simulink model "attack_decay_filter_optimized"  (R2020b)
settings: Solver=FixedStepAuto  StartTime=0.0  StopTime=stopTime  RelTol=1e-3
values from neighbouring files (symbols this model uses):
  buf_a = 65 .* ones(num_bands,1)    [modelparameters.m]
  buf_d = 65 .* ones(num_bands,1)    [modelparameters.m]
  num_bands = 8    [modelparameters.m]
libraries: simulink x1
settings Model: Creator=conno  LastModifiedBy=conno
settings DataIOCC: ReturnWorkspaceOutputs=off
settings ModelReferenceCC: ModelReferenceNumInstancesAllowed=Single

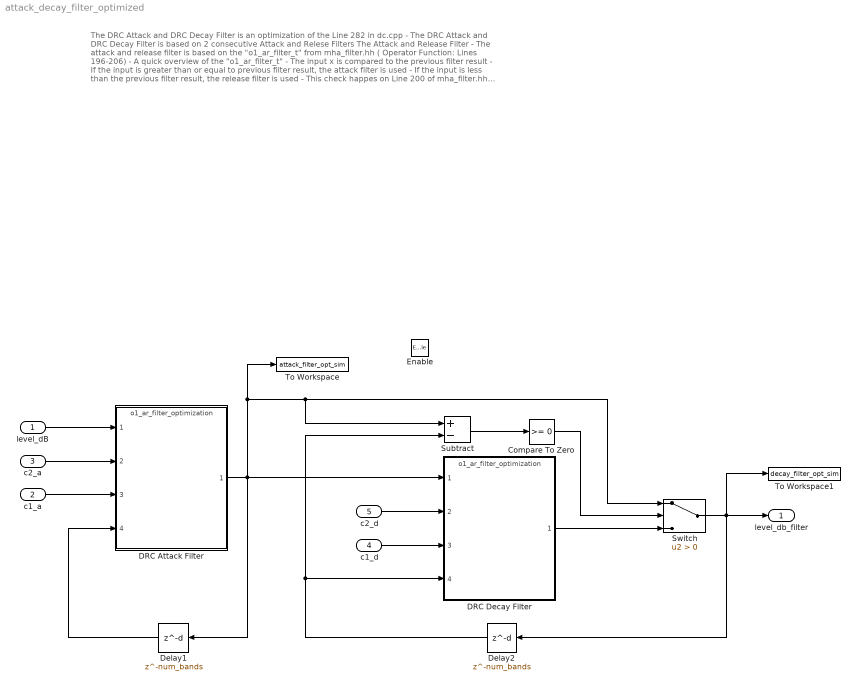
== system attack_decay_filter_optimized ==
  note: The DRC Attack and DRC Decay Filter is an optimization of the Line 282 in dc.cpp
      | - The DRC Attack and DRC Decay Filter is based on 2 consecutive Attack and Relese Filters
      | The Attack and Release Filter
      | - The attack and release filter is based on the "o1_ar_filter_t" from mha_filter.hh ( Operator Function: Lines 196-206)
      | - A quick overview of the "o1_ar_filter_t"
      | - The input x is compared to the previous filter result
      | - If the input is greater than or equal to previous filter result, the attack filter is used
      | - If the input is less than the previous filter result, the release filter is used
      | - This check happes on Line 200 of mha_filter.hh
      | Attack and Decay Filter Implementation in dc.cpp
      | - The DRC Attack Filter is a simplification of the "o1_ar_filter_t"
      | - The attack and release coefficients are the same - Lines 448-452 of mha_filter.cpp
      | - This mitigates the if statement (Line 200) of the "o1_ar_filter_t"
      | - The DRC Decay Filter is a simplifcation of the "o1_ar_filter_t" - Lines 505-509 of mha_filter.cpp
      | - The attack time constant is equal to 0
      | - c1 = 0
      | - c2 = 1
      | - The release coefficients are computed using the decay time constant
      | Simulink Optimization
      | - The DRC Attack Filter is simplified by using a single set of coefficients
      | - The result of the DRC Attack Filter is then compared to the previous result of the DRC Decay Filter
      | - If the DRC Attack Filter Result is greater than or equal, then the DRC Attack Filter Result is passed to the output
      | - Otherwise, the DRC Decay Result is passed to the output
  level_dB : Inport  OutDataTypeStr=input_type  PortDimensions=1
  c1_a : Inport  Port=2  OutDataTypeStr=ad_coeff_type  PortDimensions=1
  c2_a : Inport  Port=3  OutDataTypeStr=ad_coeff_type  PortDimensions=1
  c1_d : Inport  Port=4  OutDataTypeStr=ad_coeff_type  PortDimensions=1
  c2_d : Inport  Port=5  OutDataTypeStr=ad_coeff_type  PortDimensions=1
  Enable : EnablePort
  Compare To Zero : simulink/Logic and Bit Operations/Compare To Zero  relop=>=  OutDataTypeStr=boolean
  DRC Attack Filter : ModelReference  ModelNameDialog=o1_ar_filter_optimization.slx  SimulationMode=Normal  ModelReferenceVersion=1.152
  DRC Decay Filter : ModelReference  ModelNameDialog=o1_ar_filter_optimization.slx  SimulationMode=Normal  ModelReferenceVersion=1.152
  Delay1 : Delay  DelayLength=num_bands  InitialCondition=buf_a  UseCircularBuffer=on
  Delay2 : Delay  DelayLength=num_bands  InitialCondition=buf_d  UseCircularBuffer=on
  Subtract : Sum  Inputs=+-
  Switch : Switch  Criteria=u2 > Threshold
  To Workspace : ToWorkspace  VariableName=attack_filter_opt_sim  SampleTime=-1
  To Workspace1 : ToWorkspace  VariableName=decay_filter_opt_sim  SampleTime=-1
  level_db_filter : Outport  VectorParamsAs1DForOutWhenUnconnected=off
  wires:
  DRC Decay Filter/1 -> Switch/3
  Subtract/1 -> Compare To Zero/1
  DRC Attack Filter/1 -> DRC Decay Filter/1, Delay1/1, To Workspace/1, Subtract/1, Switch/1
  Compare To Zero/1 -> Switch/2
  Switch/1 -> To Workspace1/1, level_db_filter/1, Delay2/1
  Delay1/1 -> DRC Attack Filter/4
  Delay2/1 -> Subtract/2, DRC Decay Filter/4
  c1_a/1 -> DRC Attack Filter/3
  c2_a/1 -> DRC Attack Filter/2
  level_dB/1 -> DRC Attack Filter/1
  c2_d/1 -> DRC Decay Filter/2
  c1_d/1 -> DRC Decay Filter/3
